simulink model "Modelo_cinematico_directo"  (R2016a)
settings: Solver=FixedStepAuto  StartTime=0.0  StopTime=10.0  RelTol=1e-3
libraries: simulink x1
settings Model: Creator=daniel  LastModifiedBy=daniel
settings HardwareCC: ProdBitPerPointer=32  ProdWordSize=32  ProdHWDeviceType=Intel->x86-32 (Windows32)

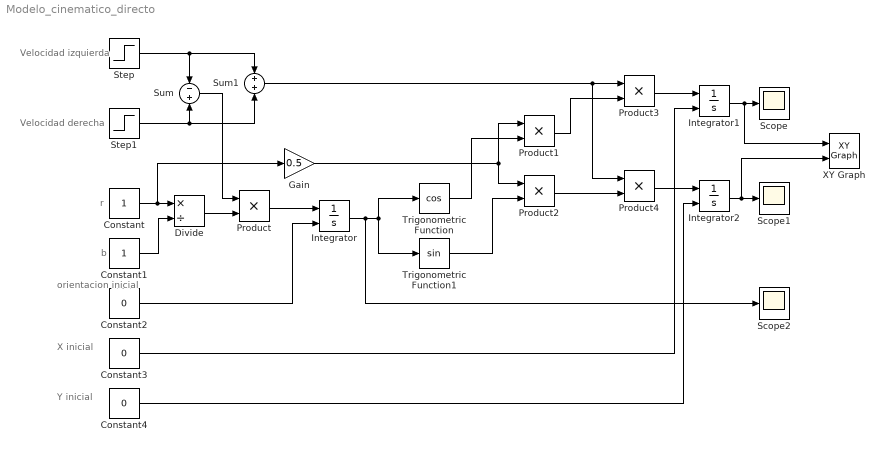
== system Modelo_cinematico_directo ==
  note: orientacion
      | inicial
  note: b
  note: r
  note: Velocidad izquierda
  note: Velocidad derecha
  note: X
      | inicial
  note: Y
      | inicial
  Constant : Constant
  Constant1 : Constant
  Constant2 : Constant  Value=0
  Constant3 : Constant  Value=0
  Constant4 : Constant  Value=0
  Divide : Product  Inputs=*/
  Gain : Gain  Gain=0.5
  Integrator : Integrator  InitialConditionSource=external
  Integrator1 : Integrator  InitialConditionSource=external
  Integrator2 : Integrator  InitialConditionSource=external
  Product{,1..4} (5 alike) : Product
  Scope : Scope
  Scope1 : Scope
  Scope2 : Scope
  Step : Step  SampleTime=0
  Step1 : Step  Time=5  SampleTime=0
  Sum : Sum  Inputs=-+
  Sum1 : Sum
  Trigonometric Function : Trigonometry  Operator=cos  OutputSignalType=real
  Trigonometric Function1 : Trigonometry  OutputSignalType=real
  XY Graph : simulink/Sinks/XY Graph  xmin=-1  xmax=1  ymin=-1  ymax=1  st=-1
  wires:
  Constant/1 -> Gain/1, Divide/1
  Constant1/1 -> Divide/2
  Divide/1 -> Product/2
  Sum/1 -> Product/1
  Product/1 -> Integrator/1
  Constant2/1 -> Integrator/2
  Integrator/1 -> Scope2/1, Trigonometric Function1/1, Trigonometric Function/1
  Trigonometric Function1/1 -> Product2/2
  Trigonometric Function/1 -> Product1/2
  Gain/1 -> Product1/1, Product2/1
  Sum1/1 -> Product4/1, Product3/1
  Product1/1 -> Product3/2
  Product2/1 -> Product4/2
  Product4/1 -> Integrator2/1
  Product3/1 -> Integrator1/1
  Integrator2/1 -> XY Graph/2, Scope1/1
  Integrator1/1 -> XY Graph/1, Scope/1
  Constant3/1 -> Integrator1/2
  Constant4/1 -> Integrator2/2
  Step1/1 -> Sum1/2, Sum/2
  Step/1 -> Sum1/1, Sum/1
